simulink model "nonlinear_controller_sim"  (R2021b)
settings: Solver=ode4  StartTime=0.0  StopTime=480.0  FixedStep=.002  RelTol=1e-3
values from neighbouring files (symbols this model uses):
  k = 1    [Inverted_Pendulum.m]    (also in si_elbow.m = k - gamma*dJdk)
settings Model: Creator=johnc  LastModifiedBy=johnc

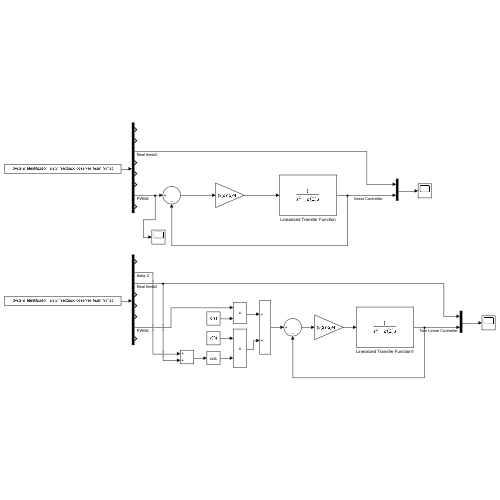
[thumbnail: Simulink's stored preview of the top-level diagram]
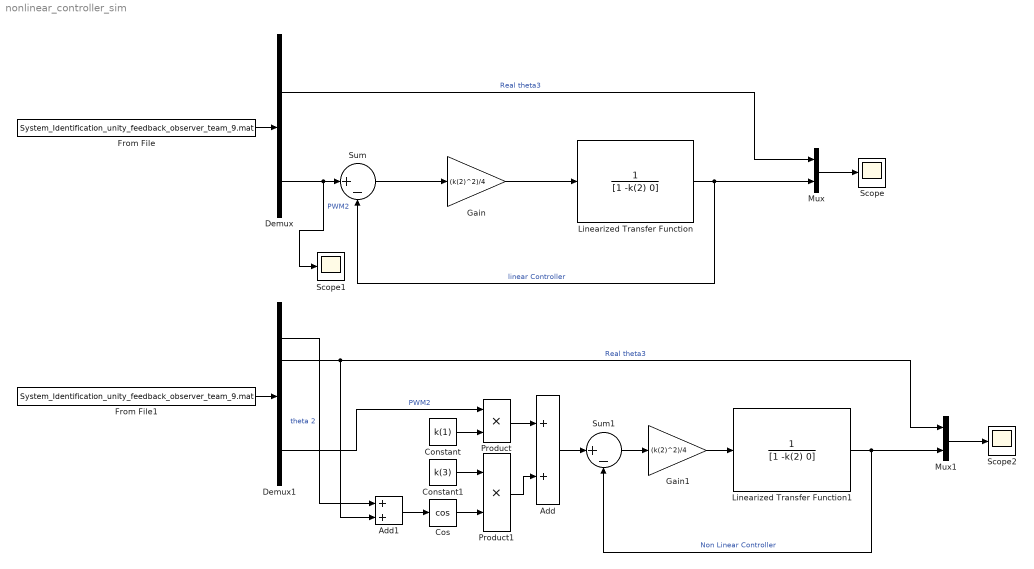
== system nonlinear_controller_sim ==
  Add : Sum
  Add1 : Sum
  Constant : Constant  Value=k(1)
  Constant1 : Constant  Value=k(3)
  Cos : Trigonometry  Operator=cos
  Demux : Demux  Outputs=8
  Demux1 : Demux  Outputs=8
  From File : FromFile  FileName=System_Identification_unity_feedback_observer_team_9.mat  SampleTime=0
  From File1 : FromFile  FileName=System_Identification_unity_feedback_observer_team_9.mat  SampleTime=0
  Gain : Gain  Gain=(k(2)^2)/4
  Gain1 : Gain  Gain=(k(2)^2)/4
  Linearized Transfer Function : TransferFcn  Denominator=[1 -k(2) 0]
  Linearized Transfer Function1 : TransferFcn  Denominator=[1 -k(2) 0]
  Mux : Mux  Inputs=2
  Mux1 : Mux  Inputs=2
  Product : Product
  Product1 : Product
  Scope : Scope
  Scope1 : Scope
  Scope2 : Scope
  Sum : Sum  Inputs=|+-
  Sum1 : Sum  Inputs=|+-
  wires:
  Gain/1 -> Linearized Transfer Function/1
  Sum/1 -> Gain/1
  From File/1 -> Demux/1
  Mux/1 -> Scope/1
  Demux/7 -> Scope1/1, Sum/1  "PWM2"
  Linearized Transfer Function/1 -> Sum/2, Mux/2  "linear Controller"
  Demux/3 -> Mux/1  "Real theta3"
  Demux1/3 -> Add1/2, Mux1/1  "Real theta3"
  Sum1/1 -> Gain1/1
  Linearized Transfer Function1/1 -> Mux1/2, Sum1/2  "Non Linear Controller"
  Mux1/1 -> Scope2/1
  From File1/1 -> Demux1/1
  Gain1/1 -> Linearized Transfer Function1/1
  Add/1 -> Sum1/1
  Product/1 -> Add/1
  Constant/1 -> Product/2
  Demux1/7 -> Product/1  "PWM2"
  Product1/1 -> Add/2
  Demux1/2 -> Add1/1  "theta 2"
  Add1/1 -> Cos/1
  Cos/1 -> Product1/2
  Constant1/1 -> Product1/1
